simulink model "model_problem2"  (R2020a)
settings: Solver=VariableStepAuto  StartTime=0.0  StopTime=10.0  RelTol=1e-3
values from neighbouring files (symbols this model uses):
  be = 2.0    [model_values.sldd]
  bv = 1.0    [model_values.sldd]
  Ie = 1.0    [model_values.sldd]
  Iv = 5.0    [model_values.sldd]
  muk = 1.0    [model_values.sldd]
  mus = 1.5    [model_values.sldd]
  R = 1.0    [model_values.sldd]
settings Model: DataDictionary=model_values.sldd  Creator=Prateek  LastModifiedBy=Prateek

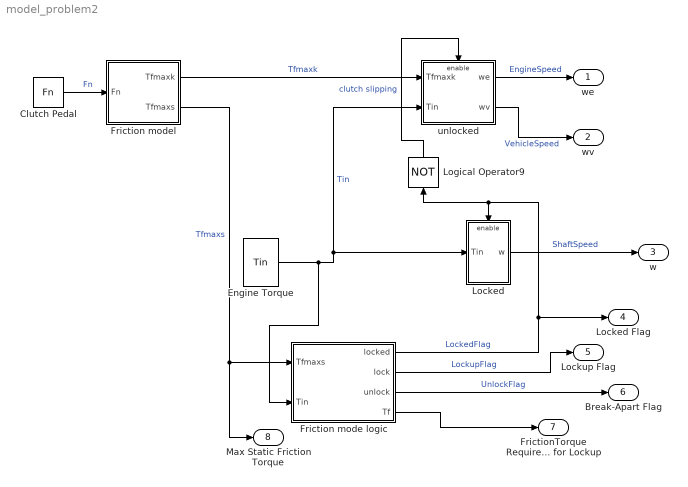
== system model_problem2 ==
  Clutch Pedal : FromWorkspace  VariableName=Fn  ZeroCross=off
  Engine Torque : FromWorkspace  VariableName=Tin  ZeroCross=off
  "Friction mode logic " : Subsystem
  Friction model : Subsystem
  Locked : Subsystem
  Logical Operator9 : Logic  Operator=NOT  Inputs=1  IconShape=distinctive  OutDataTypeStr=boolean
  unlocked : Subsystem
  we : Outport  InitialOutput=0  VectorParamsAs1DForOutWhenUnconnected=off
  wv : Outport  Port=2  InitialOutput=0  VectorParamsAs1DForOutWhenUnconnected=off
  w : Outport  Port=3  InitialOutput=0  VectorParamsAs1DForOutWhenUnconnected=off
  Locked Flag : Outport  Port=4  InitialOutput=0  VectorParamsAs1DForOutWhenUnconnected=off
  Lockup Flag : Outport  Port=5  InitialOutput=0  VectorParamsAs1DForOutWhenUnconnected=off
  Break-Apart Flag : Outport  Port=6  InitialOutput=0  VectorParamsAs1DForOutWhenUnconnected=off
  FrictionTorque Required for Lockup : Outport  Port=7  InitialOutput=0  VectorParamsAs1DForOutWhenUnconnected=off
  Max Static Friction Torque : Outport  Port=8  InitialOutput=0  VectorParamsAs1DForOutWhenUnconnected=off
  wires:
  Logical Operator9/1 -> unlocked/Enable  "clutch slipping"
  Locked/1(w) -> w/1  "ShaftSpeed"
  "Friction mode logic "/4(Tf) -> FrictionTorque Required for Lockup/1
  Clutch Pedal/1 -> Friction model/1(Fn)  "Fn"
  unlocked/1(we) -> we/1  "EngineSpeed"
  Friction model/2(Tfmaxs) -> Max Static Friction Torque/1, "Friction mode logic "/1(Tfmaxs)  "Tfmaxs"
  "Friction mode logic "/1(locked) -> Locked Flag/1, Logical Operator9/1, Locked/Enable  "LockedFlag"
  Engine Torque/1 -> "Friction mode logic "/2(Tin), unlocked/2(Tin), Locked/1(Tin)  "Tin"
  unlocked/2(wv) -> wv/1  "VehicleSpeed"
  "Friction mode logic "/2(lock) -> Lockup Flag/1  "LockupFlag"
  "Friction mode logic "/3(unlock) -> Break-Apart Flag/1  "UnlockFlag"
  Friction model/1(Tfmaxk) -> unlocked/1(Tfmaxk)  "Tfmaxk"

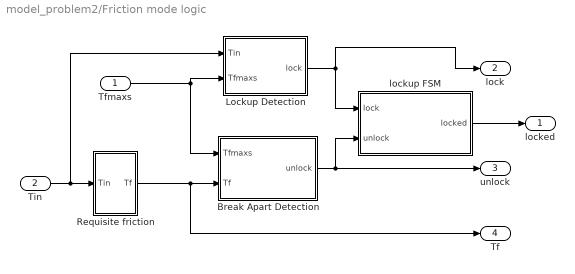
== system model_problem2/Friction mode logic  ==
  Tfmaxs : Inport
  Tin : Inport  Port=2
  Break Apart Detection : Subsystem
  Lockup Detection : Subsystem
  Requisite friction : Subsystem
  lockup FSM : Subsystem
  locked : Outport  InitialOutput=0  VectorParamsAs1DForOutWhenUnconnected=off
  lock : Outport  Port=2  InitialOutput=0  VectorParamsAs1DForOutWhenUnconnected=off
  unlock : Outport  Port=3  InitialOutput=0  VectorParamsAs1DForOutWhenUnconnected=off
  Tf : Outport  Port=4  InitialOutput=0  VectorParamsAs1DForOutWhenUnconnected=off
  wires:
  Tin/1 -> Lockup Detection/1(Tin), Requisite friction/1(Tin)
  Requisite friction/1(Tf) -> Break Apart Detection/2(Tf), Tf/1
  Tfmaxs/1 -> Lockup Detection/2(Tfmaxs), Break Apart Detection/1(Tfmaxs)
  Lockup Detection/1(lock) -> lockup FSM/1(lock), lock/1
  lockup FSM/1(locked) -> locked/1
  Break Apart Detection/1(unlock) -> lockup FSM/2(unlock), unlock/1

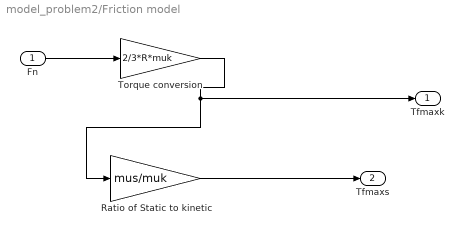
== system model_problem2/Friction model ==
  Fn : Inport
  Ratio of Static to kinetic : Gain  Gain=mus/muk  SaturateOnIntegerOverflow=on  OutDataTypeStr=Inherit: Same as input  ParamDataTypeStr=Inherit: Same as input
  Torque conversion : Gain  Gain=2/3*R*muk  SaturateOnIntegerOverflow=on  OutDataTypeStr=Inherit: Same as input  ParamDataTypeStr=Inherit: Same as input
  Tfmaxk : Outport  InitialOutput=0  VectorParamsAs1DForOutWhenUnconnected=off
  Tfmaxs : Outport  Port=2  InitialOutput=0  VectorParamsAs1DForOutWhenUnconnected=off
  wires:
  Torque conversion/1 -> Tfmaxk/1, Ratio of Static to kinetic/1
  Fn/1 -> Torque conversion/1
  Ratio of Static to kinetic/1 -> Tfmaxs/1

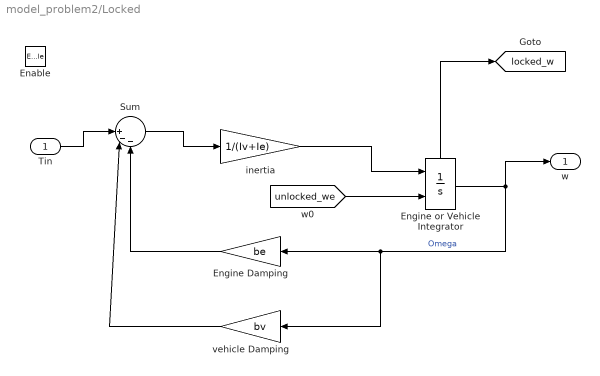
== system model_problem2/Locked ==
  Tin : Inport
  Enable : EnablePort  StatesWhenEnabling=reset
  Engine Damping : Gain  Gain=be  SaturateOnIntegerOverflow=on  OutDataTypeStr=Inherit: Same as input  ParamDataTypeStr=Inherit: Same as input
  Engine or Vehicle Integrator : Integrator  InitialConditionSource=external  ShowStatePort=on
  Sum : Sum  Inputs=||+--  InputSameDT=on  SaturateOnIntegerOverflow=on  OutDataTypeStr=Inherit: Same as first input
  inertia : Gain  Gain=1/(Iv+Ie)  SaturateOnIntegerOverflow=on  OutDataTypeStr=Inherit: Same as input  ParamDataTypeStr=Inherit: Same as input
  vehicle Damping : Gain  Gain=bv  SaturateOnIntegerOverflow=on  OutDataTypeStr=Inherit: Same as input  ParamDataTypeStr=Inherit: Same as input
  w : Outport  InitialOutput=0  VectorParamsAs1DForOutWhenUnconnected=off
  tag scope: locked_w=global
  wires:
  Engine Damping/1 -> Sum/3
  Sum/1 -> inertia/1
  inertia/1 -> Engine or Vehicle Integrator/1
  vehicle Damping/1 -> Sum/2
  Engine or Vehicle Integrator/1 -> w/1, Engine Damping/1, vehicle Damping/1  "Omega"
  [unlocked_we] -> Engine or Vehicle Integrator/2
  Tin/1 -> Sum/1
  Engine or Vehicle Integrator/State -> [locked_w]

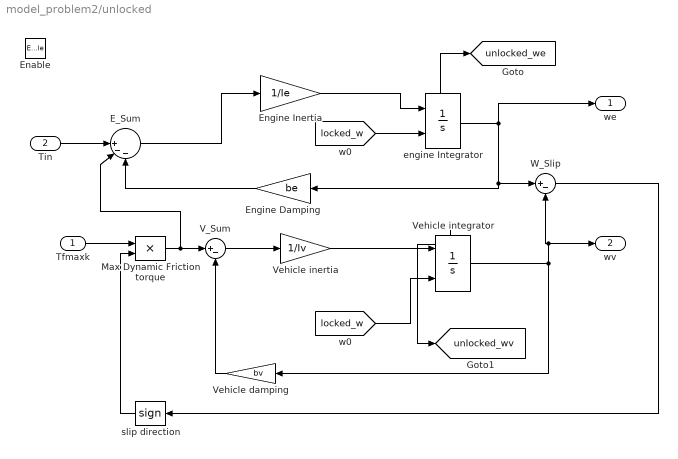
== system model_problem2/unlocked ==
  Tfmaxk : Inport
  Tin : Inport  Port=2
  Enable : EnablePort  StatesWhenEnabling=reset
  E_Sum : Sum  Inputs=||+--  InputSameDT=on  SaturateOnIntegerOverflow=on  OutDataTypeStr=Inherit: Same as first input
  Engine Damping : Gain  Gain=be  SaturateOnIntegerOverflow=on  OutDataTypeStr=Inherit: Same as input  ParamDataTypeStr=Inherit: Same as input
  Engine Inertia : Gain  Gain=1/Ie  SaturateOnIntegerOverflow=on  OutDataTypeStr=Inherit: Same as input  ParamDataTypeStr=Inherit: Same as input
  Max Dynamic Friction torque : Product  InputSameDT=on  RndMeth=Zero  SaturateOnIntegerOverflow=on  OutDataTypeStr=Inherit: Same as first input
  V_Sum : Sum  Inputs=|+-  InputSameDT=on  SaturateOnIntegerOverflow=on  OutDataTypeStr=Inherit: Same as first input
  Vehicle damping : Gain  Gain=bv  SaturateOnIntegerOverflow=on  OutDataTypeStr=Inherit: Same as input  ParamDataTypeStr=Inherit: Same as input
  Vehicle inertia : Gain  Gain=1/Iv  SaturateOnIntegerOverflow=on  OutDataTypeStr=Inherit: Same as input  ParamDataTypeStr=Inherit: Same as input
  Vehicle integrator : Integrator  InitialConditionSource=external  ShowStatePort=on
  W_Slip : Sum  Inputs=|+-  InputSameDT=on  SaturateOnIntegerOverflow=on  OutDataTypeStr=Inherit: Same as first input
  engine Integrator : Integrator  InitialConditionSource=external  ShowStatePort=on
  slip direction : Signum
  we : Outport  InitialOutput=0  VectorParamsAs1DForOutWhenUnconnected=off
  wv : Outport  Port=2  InitialOutput=0  VectorParamsAs1DForOutWhenUnconnected=off
  tag scope: unlocked_we=global, unlocked_wv=global
  wires:
  [locked_w] -> engine Integrator/2
  Engine Damping/1 -> E_Sum/3
  E_Sum/1 -> Engine Inertia/1
  engine Integrator/1 -> we/1, Engine Damping/1, W_Slip/1
  Vehicle integrator/State -> [unlocked_wv]
  Tin/1 -> E_Sum/1
  engine Integrator/State -> [unlocked_we]
  [locked_w] -> Vehicle integrator/2
  Vehicle damping/1 -> V_Sum/2
  slip direction/1 -> Max Dynamic Friction torque/2
  Vehicle integrator/1 -> Vehicle damping/1, wv/1, W_Slip/2
  Max Dynamic Friction torque/1 -> V_Sum/1, E_Sum/2
  V_Sum/1 -> Vehicle inertia/1
  Engine Inertia/1 -> engine Integrator/1
  Vehicle inertia/1 -> Vehicle integrator/1
  W_Slip/1 -> slip direction/1
  Tfmaxk/1 -> Max Dynamic Friction torque/1

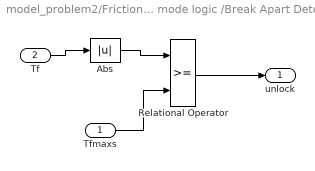
== system model_problem2/Friction mode logic /Break Apart Detection ==
  Tfmaxs : Inport
  Tf : Inport  Port=2
  Abs : Abs  SaturateOnIntegerOverflow=on
  Relational Operator : RelationalOperator  OutDataTypeStr=boolean  RndMeth=Nearest  InputSameDT=on
  unlock : Outport  InitialOutput=0  VectorParamsAs1DForOutWhenUnconnected=off
  wires:
  Relational Operator/1 -> unlock/1
  Tfmaxs/1 -> Relational Operator/2
  Abs/1 -> Relational Operator/1
  Tf/1 -> Abs/1

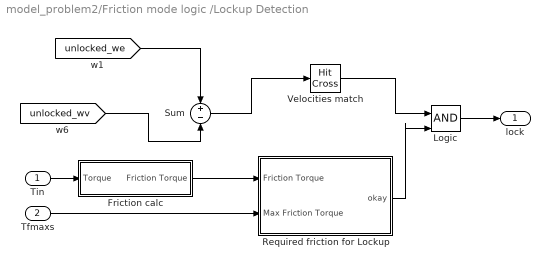
== system model_problem2/Friction mode logic /Lockup Detection ==
  Tin : Inport
  Tfmaxs : Inport  Port=2
  Friction calc : Subsystem
  Logic : Logic  IconShape=distinctive  OutDataTypeStr=boolean
  Required friction for Lockup : Subsystem
  Sum : Sum  Inputs=+-  InputSameDT=on  SaturateOnIntegerOverflow=on  OutDataTypeStr=Inherit: Same as first input
  Velocities match : HitCross
  lock : Outport  InitialOutput=0  VectorParamsAs1DForOutWhenUnconnected=off
  wires:
  Tfmaxs/1 -> Required friction for Lockup/2(Max Friction Torque)
  Required friction for Lockup/1(okay) -> Logic/2
  Friction calc/1(Friction Torque) -> Required friction for Lockup/1(Friction Torque)
  Tin/1 -> Friction calc/1(Torque)
  [unlocked_wv] -> Sum/2
  Velocities match/1 -> Logic/1
  Sum/1 -> Velocities match/1
  Logic/1 -> lock/1
  [unlocked_we] -> Sum/1

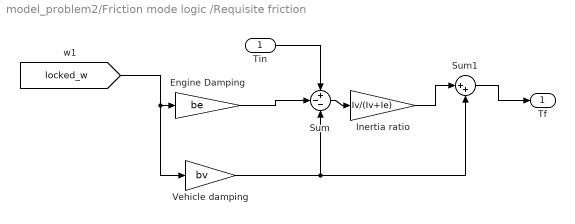
== system model_problem2/Friction mode logic /Requisite friction ==
  Tin : Inport
  Engine Damping : Gain  Gain=be  SaturateOnIntegerOverflow=on  OutDataTypeStr=Inherit: Same as input  ParamDataTypeStr=Inherit: Same as input
  Inertia ratio : Gain  Gain=Iv/(Iv+Ie)  SaturateOnIntegerOverflow=on  OutDataTypeStr=Inherit: Same as input  ParamDataTypeStr=Inherit: Same as input
  Sum : Sum  Inputs=+--  InputSameDT=on  SaturateOnIntegerOverflow=on  OutDataTypeStr=Inherit: Same as first input
  Sum1 : Sum  Inputs=|++  InputSameDT=on  SaturateOnIntegerOverflow=on  OutDataTypeStr=Inherit: Same as first input
  Vehicle damping : Gain  Gain=bv  SaturateOnIntegerOverflow=on  OutDataTypeStr=Inherit: Same as input  ParamDataTypeStr=Inherit: Same as input
  Tf : Outport  InitialOutput=0  VectorParamsAs1DForOutWhenUnconnected=off
  wires:
  Sum1/1 -> Tf/1
  Vehicle damping/1 -> Sum/3, Sum1/2
  [locked_w] -> Vehicle damping/1, Engine Damping/1
  Engine Damping/1 -> Sum/2
  Tin/1 -> Sum/1
  Inertia ratio/1 -> Sum1/1
  Sum/1 -> Inertia ratio/1

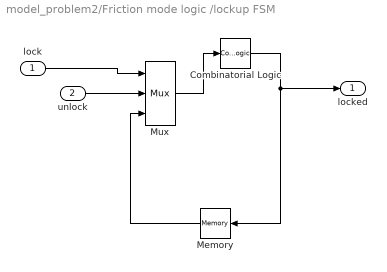
== system model_problem2/Friction mode logic /lockup FSM ==
  lock : Inport
  unlock : Inport  Port=2
  Combinatorial Logic : CombinatorialLogic  TruthTable=[0;1;0;0;1;1;1;0]
  Memory : Memory
  Mux : Mux  Inputs=3
  locked : Outport  InitialOutput=0  VectorParamsAs1DForOutWhenUnconnected=off
  wires:
  lock/1 -> Mux/1
  Combinatorial Logic/1 -> locked/1, Memory/1
  Memory/1 -> Mux/3
  Mux/1 -> Combinatorial Logic/1
  unlock/1 -> Mux/2

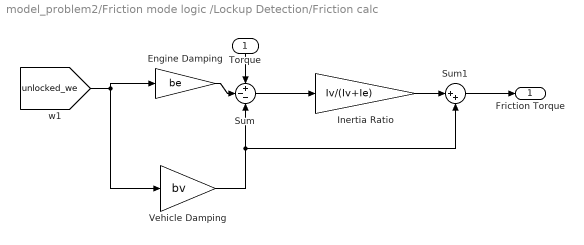
== system model_problem2/Friction mode logic /Lockup Detection/Friction calc ==
  Torque : Inport
  Engine Damping : Gain  Gain=be  SaturateOnIntegerOverflow=on  OutDataTypeStr=Inherit: Same as input  ParamDataTypeStr=Inherit: Same as input
  Inertia Ratio : Gain  Gain=Iv/(Iv+Ie)  SaturateOnIntegerOverflow=on  OutDataTypeStr=Inherit: Same as input  ParamDataTypeStr=Inherit: Same as input
  Sum : Sum  Inputs=+--  InputSameDT=on  SaturateOnIntegerOverflow=on  OutDataTypeStr=Inherit: Same as first input
  Sum1 : Sum  Inputs=|++  InputSameDT=on  SaturateOnIntegerOverflow=on  OutDataTypeStr=Inherit: Same as first input
  Vehicle Damping : Gain  Gain=bv  SaturateOnIntegerOverflow=on  OutDataTypeStr=Inherit: Same as input  ParamDataTypeStr=Inherit: Same as input
  Friction Torque : Outport  InitialOutput=0  VectorParamsAs1DForOutWhenUnconnected=off
  wires:
  [unlocked_we] -> Vehicle Damping/1, Engine Damping/1
  Vehicle Damping/1 -> Sum1/2, Sum/3
  Engine Damping/1 -> Sum/2
  Sum/1 -> Inertia Ratio/1
  Torque/1 -> Sum/1
  Inertia Ratio/1 -> Sum1/1
  Sum1/1 -> Friction Torque/1

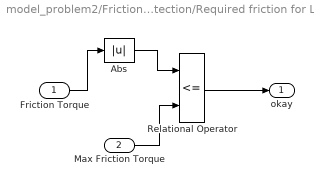
== system model_problem2/Friction mode logic /Lockup Detection/Required friction for Lockup ==
  Friction Torque : Inport
  Max Friction Torque : Inport  Port=2
  Abs : Abs  SaturateOnIntegerOverflow=on
  Relational Operator : RelationalOperator  Operator=<=  OutDataTypeStr=boolean  RndMeth=Nearest  InputSameDT=on
  okay : Outport  InitialOutput=0  VectorParamsAs1DForOutWhenUnconnected=off
  wires:
  Friction Torque/1 -> Abs/1
  Relational Operator/1 -> okay/1
  Abs/1 -> Relational Operator/1
  Max Friction Torque/1 -> Relational Operator/2
